simulink model "LCC_S"  (R2020a)
settings: Solver=VariableStepAuto  StartTime=0.0  StopTime=10e-3  RelTol=1e-3
libraries: powerlib x27, eeRmsMeasurement x7
settings Model: Creator=赵健  LastModifiedBy=赵健

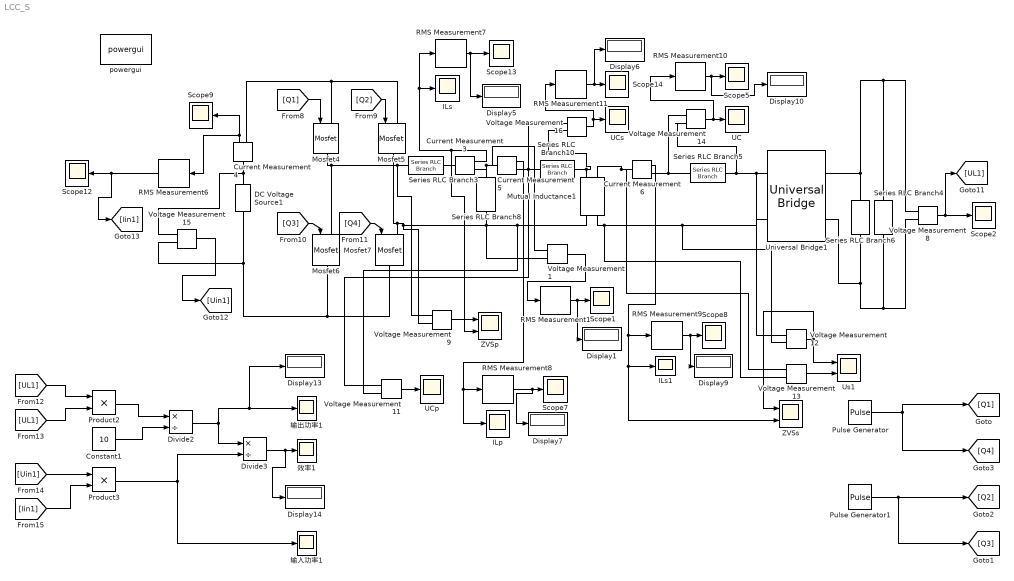
== system LCC_S ==
  Constant1 : Constant  Value=10
  Current Measurement{3..6} (4 alike) : powerlib/Measurements/Current Measurement  PhasorSimulation=off  OutputType=Complex  PSBequivalent=0
  DC Voltage Source1 : powerlib/Electrical Sources/DC Voltage Source  Amplitude=15  Measurements=None
  Display{1,5..7,9..10,13..14} (8 alike) : Display
  Divide2 : Product  Inputs=*/
  Divide3 : Product  Inputs=*/
  ILp : Scope
  ILs : Scope
  ILs1 : Scope
  Mosfet{4..7} (4 alike) : powerlib/Power Electronics/Mosfet  Ron=0.044  Lon=0  Rd=0.01  Vfd=0  IC=0  Rs=1e5  Cs=inf  Measurements=off
  Mutual Inductance1 : powerlib/Elements/Mutual Inductance  LConnTagsString=a|b  RConnTagsString=A|B  TypeOfMutual=Two or three windings with equal mutual terms  NumberOfWindings=3  SelfImpedance1=[0.05 30e-6]  SelfImpedance2=[0.05 14e-6]  ThreeWindings=off  SelfImpedance3=[ 1.1 1.1e-03]  MutualImpedance=[0 5e-6]  InductanceMatrix="[1.0 0.9  0.9 ;  0.9 1.0  0.9;  0.9 0.9 1.0 ] * 1e-3"  ResistanceMatrix="[1.0 0.9  0.9 ;  0.9 1.0  0.9;  0.9 0.9 1.0 ]"  Measurements=None
      settings: AttributesFormatString=\n  SourceProductBaseCode=PS
  Product2 : Product
  Product3 : Product
  Pulse Generator : DiscretePulseGenerator  PulseType=Time based  Period=1/100000  PulseWidth=50
  Pulse Generator1 : DiscretePulseGenerator  PulseType=Time based  Period=1/100000  PulseWidth=50  PhaseDelay=1/200000
  RMS Measurement{1,6..11} (7 alike) : eeRmsMeasurement/RMS Measurement  LabelModeActiveChoice=Total  F=100000  SpecifyHarmonics=off  K=[0 1 2]  Ts=0
      settings: SourceProductBaseCode=PS
  Scope{1..2,5,7..9,12..14} (9 alike) : Scope
  Series RLC Branch10 : powerlib/Elements/Series RLC Branch  LConnTagsString=__new0  RConnTagsString=__new0  BranchType=C  Resistance=0.034  Inductance=1e-3  SetiL0=off  InitialCurrent=0  Capacitance=100.12e-9  Setx0=off  InitialVoltage=0  Measurements=None
  Series RLC Branch3 : powerlib/Elements/Series RLC Branch  LConnTagsString=__new0  RConnTagsString=__new0  BranchType=L  Resistance=1  Inductance=4.7e-6  SetiL0=off  InitialCurrent=0  Capacitance=100e-9  Setx0=off  InitialVoltage=0  Measurements=None
  Series RLC Branch4 : powerlib/Elements/Series RLC Branch  LConnTagsString=__new0  RConnTagsString=__new0  BranchType=R  Resistance=10  Inductance=1e-3  SetiL0=off  InitialCurrent=0  Capacitance=1e-6  Setx0=off  InitialVoltage=0  Measurements=None
  Series RLC Branch5 : powerlib/Elements/Series RLC Branch  LConnTagsString=__new0  RConnTagsString=__new0  BranchType=C  Resistance=0.023  Inductance=1e-3  SetiL0=off  InitialCurrent=0  Capacitance=180.93e-9  Setx0=off  InitialVoltage=0  Measurements=None
  Series RLC Branch6 : powerlib/Elements/Series RLC Branch  LConnTagsString=__new0  RConnTagsString=__new0  BranchType=C  Resistance=20  Inductance=1e-3  SetiL0=off  InitialCurrent=0  Capacitance=470e-6  Setx0=off  InitialVoltage=0  Measurements=None
  Series RLC Branch8 : powerlib/Elements/Series RLC Branch  LConnTagsString=__new0  RConnTagsString=__new0  BranchType=C  Resistance=0.023  Inductance=1e-3  SetiL0=off  InitialCurrent=0  Capacitance=538.94e-9  Setx0=off  InitialVoltage=0  Measurements=None
  UC : Scope
  UCp : Scope
  UCs : Scope
  Universal Bridge1 : powerlib/Power Electronics/Universal Bridge  Arms=2  SnubberResistance=1e5  SnubberCapacitance=inf  Device=Diodes  Ron=1e-3  Lon=0  ForwardVoltages="[  0  0  ]"  ForwardVoltage=0  GTOparameters=[ 10e-6 , 20e-6 ]  IGBTparameters=[ 1e-6 , 2e-6 ]  Measurements=None  Measurements_2=None  converterType=Rectifier
  Us1 : Scope  NumInputPorts=2
  Voltage Measurement{1,8..9,11..16} (9 alike) : powerlib/Measurements/Voltage Measurement  PhasorSimulation=off  OutputType=Complex  PSBequivalent=0
  ZVSp : Scope  NumInputPorts=2
  ZVSs : Scope  NumInputPorts=2
  powergui : powerlib/powergui  Priority=1  SimulationMode=Discrete  SampleTime=1e-8  frequency=60  Iterations=50  frequencyindice=0  Pbase=100e6  ErrMax=1e-4  UnitsV=kV  UnitsW=MW  buscounter=0  FunctionMessages=off  echomessages=off  EnableUseOfTLC=off  CurrentSourceSwitches=off  DisableSnubberDevices=off  DisableRonSwitches=off  DisableVfSwitches=off  DisplayEquations=off  AutomaticDiscreteSolvers=off  SolverType=Tustin/Backward Euler (TBE)  Interpol=off  ExternalGateDelay=off  methode=off  Ts=10  x0status=blocks  SPID=off  SwTol=0  HookPort=off  NonlinearTolerance=0  nMaxIteration=15  ContinueOnMaxIteration=off  RestoreLinks=warning  ResistiveCurrentMeasurement=off  Frange=[0:2:500]  Ylog=off  Xlog=on  ShowGrid=off  save=off  variable=ZData  structure=0  ZoomFFT=off  StartTime=0.0  cycles=1  DisplayStyle=1  fundamental=60  FreqAxis=off  MaxFrequency=1000  frequencyindicesteady=1  RmsSteady=1  display=off
  效率1 : Scope
  输入功率1 : Scope
  输出功率1 : Scope
  wires:
  Divide2/1 -> Display13/1, 输出功率1/1, Divide3/1
  Voltage Measurement15/1 -> [Uin1]
  RMS Measurement8/1 -> Display7/1, Scope7/1
  [UL1] -> Product2/1
  [Q4] -> Mosfet7/1
  RMS Measurement9/1 -> Display9/1, Scope8/1
  [Iin1] -> Product3/2
  Current Measurement4/1 -> Scope9/1, RMS Measurement6/1
  Voltage Measurement14/1 -> RMS Measurement10/1, UC/1
  [Q1] -> Mosfet4/1
  Current Measurement6/1 -> ZVSs/2, ILs1/1, RMS Measurement9/1
  Voltage Measurement8/1 -> [UL1], Scope2/1
  Voltage Measurement9/1 -> ZVSp/1
  Voltage Measurement12/1 -> ZVSs/1, Us1/1
  Pulse Generator1/1 -> [Q3], [Q2]
  Pulse Generator/1 -> [Q1], [Q4]
  Current Measurement5/1 -> ILp/1, RMS Measurement8/1
  RMS Measurement7/1 -> Display5/1, Scope13/1
  [Q2] -> Mosfet5/1
  Current Measurement3/1 -> ZVSp/2, ILs/1, RMS Measurement7/1
  Voltage Measurement16/1 -> UCs/1, RMS Measurement11/1
  [Uin1] -> Product3/1
  RMS Measurement6/1 -> [Iin1], Scope12/1
  RMS Measurement11/1 -> Display6/1, Scope14/1
  Product3/1 -> 输入功率1/1, Divide3/2
  Divide3/1 -> Display14/1, 效率1/1
  RMS Measurement10/1 -> Display10/1, Scope5/1
  Voltage Measurement13/1 -> Us1/2
  [Q3] -> Mosfet6/1
  Product2/1 -> Divide2/1
  Constant1/1 -> Divide2/2
  [UL1] -> Product2/2
  Voltage Measurement11/1 -> UCp/1
  RMS Measurement1/1 -> Display1/1, Scope1/1
  Voltage Measurement1/1 -> RMS Measurement1/1
  connections:
  Current Measurement6/LConn1 -- Voltage Measurement13/LConn1 -- Mutual Inductance1/LConn2
  Mosfet4/RConn1 -- Mosfet6/LConn1 -- Series RLC Branch3/LConn1 -- Voltage Measurement9/LConn1
  DC Voltage Source1/LConn1 -- Mosfet7/RConn1 -- Mosfet6/RConn1 -- Voltage Measurement15/LConn2
  Voltage Measurement9/LConn2 -- Mosfet5/RConn1 -- Mosfet7/LConn1 -- Voltage Measurement1/LConn2 -- Series RLC Branch8/RConn1 -- Voltage Measurement11/LConn2 -- Mutual Inductance1/RConn1
  Series RLC Branch8/LConn1 -- Voltage Measurement1/LConn1 -- Current Measurement5/LConn1 -- Current Measurement3/RConn1
  Voltage Measurement12/LConn2 -- Voltage Measurement13/LConn2 -- Mutual Inductance1/RConn2 -- Universal Bridge1/LConn2
  Voltage Measurement12/LConn1 -- Series RLC Branch5/RConn1 -- Voltage Measurement14/LConn2 -- Universal Bridge1/LConn1
  Voltage Measurement14/LConn1 -- Current Measurement6/RConn1 -- Series RLC Branch5/LConn1
  Current Measurement4/RConn1 -- Mosfet5/LConn1 -- Mosfet4/LConn1
  Voltage Measurement15/LConn1 -- DC Voltage Source1/RConn1 -- Current Measurement4/LConn1
  Series RLC Branch6/RConn1 -- Voltage Measurement8/LConn2 -- Series RLC Branch4/RConn1 -- Universal Bridge1/RConn2
  Universal Bridge1/RConn1 -- Series RLC Branch6/LConn1 -- Voltage Measurement8/LConn1 -- Series RLC Branch4/LConn1
  Voltage Measurement16/LConn2 -- Series RLC Branch10/RConn1 -- Mutual Inductance1/LConn1
  Current Measurement3/LConn1 -- Series RLC Branch3/RConn1
  Voltage Measurement11/LConn1 -- Series RLC Branch10/LConn1 -- Voltage Measurement16/LConn1 -- Current Measurement5/RConn1
